simulink subsystem "analogInputs"  (R2022b)
settings: Solver=VariableStepAuto  StartTime=0.0  StopTime=10.0  RelTol=1e-3
libraries: pot_test x1
settings Model: Creator=serga  LastModifiedBy=serga

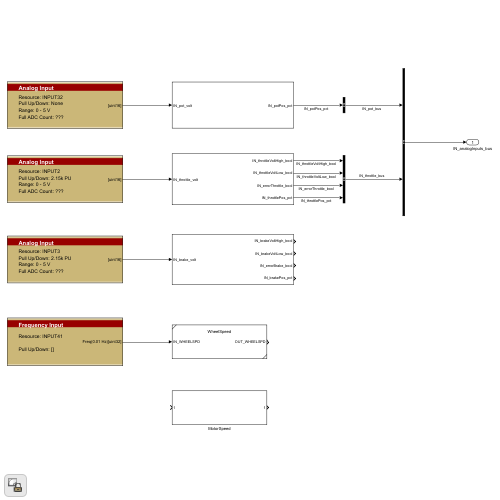
[thumbnail: Simulink's stored preview of the top-level diagram]
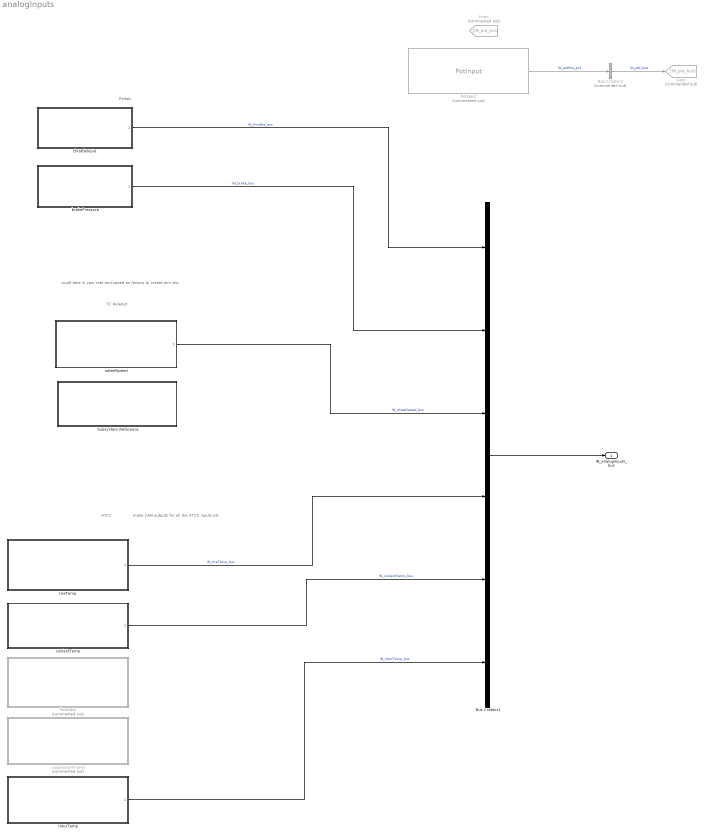
== system analogInputs ==
  note: could take in yaw rate and speed as factors to create aim slip
  note: make CAN outputs for all the ATCC inputs pls
  note: Pedals
  note: TC Related
  note: ATCC
  Bus Creator1 : BusCreator  Inputs=6
  Bus Creator2 : BusCreator  Commented=on  Inputs=1
  From : From  Commented=on  GotoTag=IN_pot_bus
  Goto : Goto  Commented=on  GotoTag=IN_pot_bus
  PotInput : pot_test/PotInput  Commented=on  SystemSampleTime=-1  VariantActivationTime=update diagram  Latency=0  AutoFrameSizeCalculation=off
  Subsystem Reference : Subsystem  ReferencedSubsystem=tcDial
  brakePressure : Subsystem  ReferencedSubsystem=brakePressure
  coolantTemp : Subsystem  ReferencedSubsystem=coolantTemp
  flowRate : Subsystem  Commented=on  ReferencedSubsystem=flowRate
  rotorTemp : Subsystem  ReferencedSubsystem=rotorTemp
  suspensionTravel : Subsystem  Commented=on  ReferencedSubsystem=suspensionTravel
  throttleInput : Subsystem  ReferencedSubsystem=throttleInput
  tireTemp : Subsystem  ReferencedSubsystem=tireTemp
  wheelSpeed : Subsystem  ReferencedSubsystem=wheelSpeed
  IN_analogInputs_bus : Outport
  wires:
  Bus Creator1/1 -> IN_analogInputs_bus/1
  PotInput/1 -> Bus Creator2/1  "IN_potPos_pct"
  Bus Creator2/1 -> Goto/1  "IN_pot_bus"
  throttleInput/1 -> Bus Creator1/1  "IN_throttle_bus"
  brakePressure/1 -> Bus Creator1/2  "IN_brake_bus"
  wheelSpeed/1 -> Bus Creator1/3  "IN_wheelSpeed_bus"
  rotorTemp/1 -> Bus Creator1/6  "IN_rotorTemp_bus"
  tireTemp/1 -> Bus Creator1/4  "IN_tireTemp_bus"
  coolantTemp/1 -> Bus Creator1/5  "IN_coolantTemp_bus"
